simulink model "ieee_80211b_rx"  (R2018a)
settings: Solver=FixedStepDiscrete  StartTime=0.0  StopTime=length(rcvd.signals.values)*(p80211.SamplesPerChannelFrame / (p80211.ChipRate*p80211.SamplesPerChip))  RelTol=1e-3
InitFcn:
  | init;
  | load('data', 'rcvd');
model workspace: external: MAT-File (data not in the file)
values from neighbouring files (symbols this model uses):
  p80211 = commwlan80211BeaconRxInit(agcStepSize, agcMaxGain,      corrThreshold, sampsPerChip)    [wlan80211BeaconRxModelParams.m]
libraries: commwlan80211BeaconLib x3, commsync2 x2, dspsigops x2, commdigbbndpm3 x1, commsequence2 x1, dspnetwork x1, commrfcorlib x1, commfilt2 x1
Description:
  | IEEE 802.11 WLAN Beacon Frame Receiver for Captured Data
  | 
  | This example shows how to process a captured beacon frame and display the
  | frame information.
settings Model: Creator=The MathWorks, Inc.  LastModifiedBy=tung
settings DataIOCC: LimitDataPoints=on  SaveFormat=Array  SaveOutput=off  SignalLogging=off  DSMLogging=off  SaveTime=off
settings OptimizationCC: DefaultParameterBehavior=Inlined  InlineInvariantSignals=on  ExpressionDepthLimit=2147483647  EfficientFloat2IntCast=on  LifeSpan=inf
settings DebuggingCC: UnderspecifiedInitializationDetection=Classic  MergeDetectMultiDrivingBlocksExec=none  SolverPrmCheckMsg=warning  UniqueDataStoreMsg=error  AllowSymbolicDim=off  StateNameClashWarn=warning  SFUnexpectedBacktrackingDiag=warning  SFNoUnconditionalDefaultTransitionDiag=warning  SFExecutionAtInitializationDiag=none
settings HardwareCC: ProdBitPerPointer=32  ProdBitPerSizeT=32  ProdBitPerPtrDiffT=32  ProdLargestAtomicFloat=None  ProdIntDivRoundTo=Undefined  ProdEndianess=Unspecified  ProdWordSize=32  ProdHWDeviceType=32-bit Generic
settings ModelReferenceCC: PropagateSignalLabelsOutOfModel=off
settings CodeAppCC: StateflowObjectComments=on
settings GRTTargetCC: TargetLangStandard=C89/C90 (ANSI)  GeneratePreprocessorConditionals=Disable all  CombineOutputUpdateFcns=off  GRTInterface=on
settings ConfigComp: CovMetricSettings=dw  CovHtmlReporting=on  CovSaveCumulativeToWorkspaceVar=on  CovSaveSingleToWorkspaceVar=on  CovShowResultsExplorer=off  CovExternalEMLEnable=off  CovSFcnEnable=off

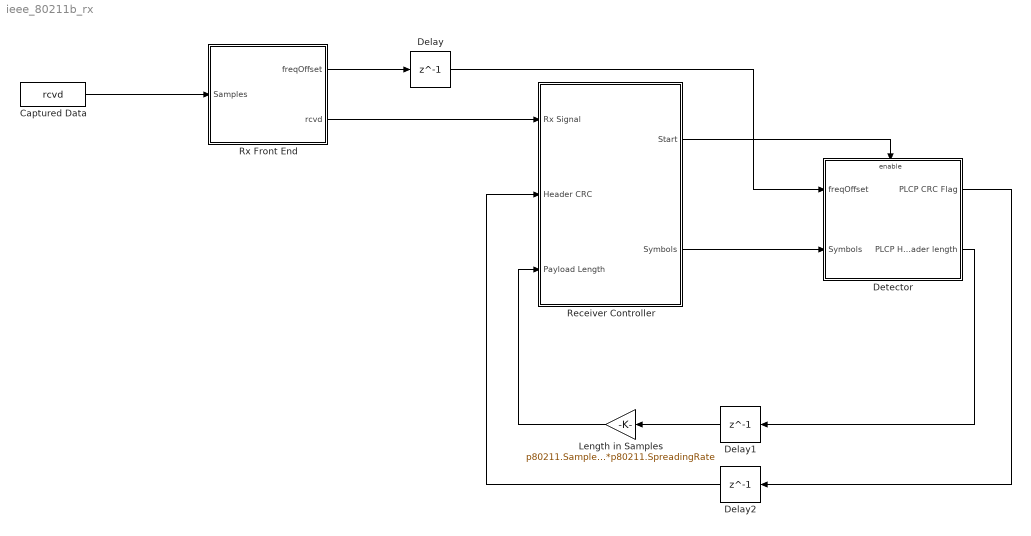
== system ieee_80211b_rx ==
  Captured Data : FromWorkspace  VariableName=rcvd  SampleTime=p80211.SamplesPerChannelFrame / (p80211.ChipRate*p80211.SamplesPerChip)  Interpolate=off  OutputAfterFinalValue=Cyclic repetition
  Delay : Delay  DelayLength=1  InitialCondition=0  InputProcessing=Columns as channels (frame based)
  Delay1 : Delay  DelayLength=1  InitialCondition=0  InputProcessing=Columns as channels (frame based)
  Delay2 : Delay  DelayLength=1  InitialCondition=0  InputProcessing=Columns as channels (frame based)
  Detector : Subsystem
      settings: CloseFcn=clear BeaconFrameBodyType rcvd
  Length in Samples : Gain  Gain=p80211.SamplesPerChip*p80211.SpreadingRate  OutDataTypeStr=uint32  SaturateOnIntegerOverflow=on  ParamDataTypeStr=Inherit: Same as input
  Receiver Controller : Subsystem
  Rx Front End : Subsystem
  wires:
  Length in Samples/1 -> Receiver Controller/3(Payload Length)
  Detector/1(PLCP CRC Flag) -> Delay2/1
  Delay2/1 -> Receiver Controller/2(Header CRC)
  Receiver Controller/1(Start) -> Detector/Enable
  Rx Front End/2(rcvd) -> Receiver Controller/1(Rx Signal)
  Delay1/1 -> Length in Samples/1
  Receiver Controller/2(Symbols) -> Detector/2(Symbols)
  Captured Data/1 -> Rx Front End/1(Samples)
  Detector/2(PLCP Header length) -> Delay1/1
  Rx Front End/1(freqOffset) -> Delay/1
  Delay/1 -> Detector/1(freqOffset)

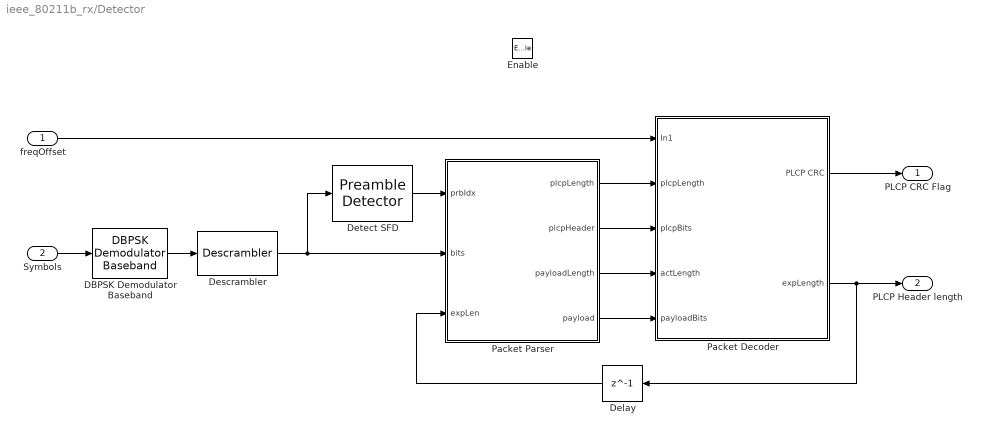
== system ieee_80211b_rx/Detector ==
  freqOffset : Inport
  Symbols : Inport  Port=2
  Enable : EnablePort  StatesWhenEnabling=reset  PropagateVarSize=During execution
  DBPSK Demodulator Baseband : commdigbbndpm3/DBPSK Demodulator Baseband  Ph=0  outDtype=Smallest unsigned integer
      settings: SourceProductName=Communications System Toolbox  SourceProductBaseCode=CM
  Delay : Delay  DelayLength=1  InitialCondition=0  InputProcessing=Columns as channels (frame based)
  Descrambler : commsequence2/Descrambler  M=2  poly=p80211.ScramblerPolynomial  iniStaSource=Dialog Parameter  ini_sta=[0 0 0 0 0 0 0]  resetViaPort=off
      settings: SourceProductName=Communications System Toolbox  SourceProductBaseCode=CM
  Detect SFD : commsync2/Preamble Detector  Input=Bit  Preamble=p80211.SFD  Threshold=3  DetectionMetricOutput=off  Detections=All  SimulateUsing=Code generation
      settings: SourceProductName=Communications System Toolbox  SourceProductBaseCode=CM
  Packet Decoder : Subsystem
  Packet Parser : MATLAB Function  TreatAsAtomicUnit=on
  PLCP CRC Flag : Outport  InitialOutput=1
  PLCP Header length : Outport  Port=2  InitialOutput=1
  wires:
  Delay/1 -> Packet Parser/3(expLen)
  Symbols/1 -> DBPSK Demodulator Baseband/1
  DBPSK Demodulator Baseband/1 -> Descrambler/1
  Detect SFD/1 -> Packet Parser/1(prbIdx)
  Descrambler/1 -> Detect SFD/1, Packet Parser/2(bits)
  Packet Decoder/1(PLCP CRC) -> PLCP CRC Flag/1
  Packet Decoder/2(expLength) -> Delay/1, PLCP Header length/1
  Packet Parser/1(plcpLength) -> Packet Decoder/2(plcpLength)
  Packet Parser/2(plcpHeader) -> Packet Decoder/3(plcpBits)
  Packet Parser/3(payloadLength) -> Packet Decoder/4(actLength)
  Packet Parser/4(payload) -> Packet Decoder/5(payloadBits)
  freqOffset/1 -> Packet Decoder/1(In1)

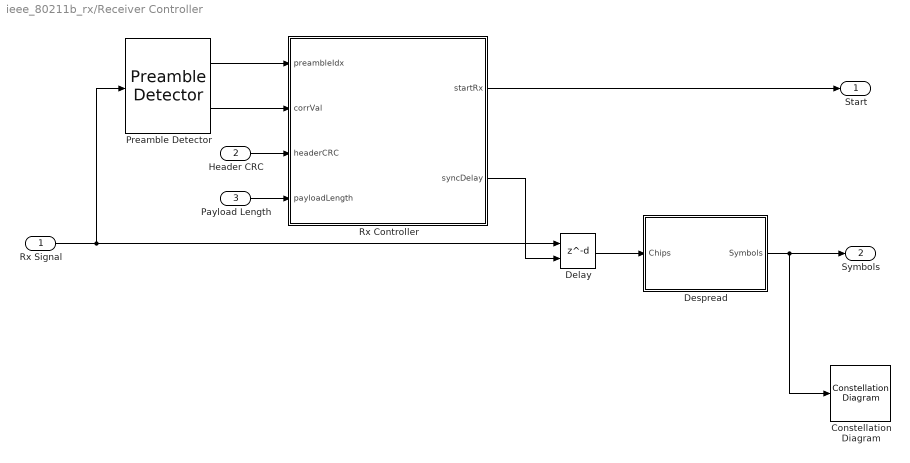
== system ieee_80211b_rx/Receiver Controller ==
  Rx Signal : Inport
  Header CRC : Inport  Port=2
  Payload Length : Inport  Port=3
  Constellation Diagram : ConstellationDiagram
  Delay : Delay  DelayLengthSource=Input port  DelayLengthUpperLimit=p80211.SamplesPerChannelFrame  InputProcessing=Columns as channels (frame based)
      settings: InputPortMap=u0,p1
  Despread : Subsystem
  Preamble Detector : commsync2/Preamble Detector  Input=Symbol  Preamble=p80211.SynchronizationSignal  Threshold=p80211.CorrelationThreshold  DetectionMetricOutput=on  Detections=All  SimulateUsing=Code generation
      settings: SourceProductName=Communications System Toolbox  SourceProductBaseCode=CM
  Rx Controller : MATLAB Function  TreatAsAtomicUnit=on
  Start : Outport
  Symbols : Outport  Port=2
  wires:
  Despread/1(Symbols) -> Constellation Diagram/1, Symbols/1
  Rx Controller/2(syncDelay) -> Delay/2
  Rx Controller/1(startRx) -> Start/1
  Header CRC/1 -> Rx Controller/3(headerCRC)
  Rx Signal/1 -> Preamble Detector/1, Delay/1
  Payload Length/1 -> Rx Controller/4(payloadLength)
  Delay/1 -> Despread/1(Chips)
  Preamble Detector/2 -> Rx Controller/2(corrVal)
  Preamble Detector/1 -> Rx Controller/1(preambleIdx)

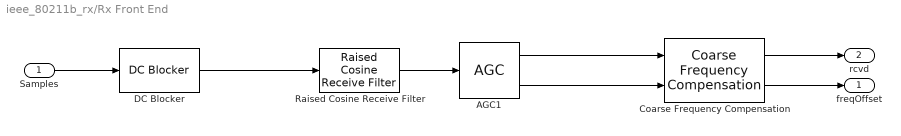
== system ieee_80211b_rx/Rx Front End ==
  Samples : Inport
  AGC1 : commrfcorlib/AGC  LegacyMode=off  DetectorMethod=Rectifier  LoopMethod=Linear  UpdatePeriod=100  StepSize=0.1  AdaptationStepSize=p80211.AGCStepSize  DesiredOutputPower=1  AveragingLength=50  MaximumGain=30  MaxPowerGain=p80211.AGCUpperLimit  GainOutputPort=off  InputPowerOutputPort=on  SimulateUsing=Code generation
      settings: SourceProductName=Communications System Toolbox
  Coarse Frequency Compensation : commwlan80211BeaconLib/Coarse Frequency Compensation  decimRate=44*p80211.SamplesPerChip/2  maxOffset=50000  M=2
      settings: SourceProductName=Communications System Toolbox  SourceProductBaseCode=CM
  DC Blocker : dspsigops/DC Blocker  Algorithm=IIR  NormalizedBandwidth=0.001  Length=8  Order=6  SimulateUsing=Code generation
      settings: SourceProductName=DSP System Toolbox  SourceProductBaseCode=DS
  Raised Cosine Receive Filter : commfilt2/Raised Cosine Receive Filter  filtType=Square root  R=0.3  filtSpan=p80211.FilterOrder  N=p80211.SamplesPerChip  downFactor=1  downOffset=0  filterGain=1  InputProcessing=Columns as channels (frame based)  RateOptions=Enforce single-rate processing  framing=Mute  checkCoeff=off  variableName=rcRxFilt  currentFiltSpan=2*(p80211.FilterOrder/2)  D=p80211.FilterOrder/2  inputOffset=0  sampMode=Mute  saveAsFlag=0  rateMode=Downsampling  checkGain=Normalized  launchFVT=off  roundingMode=Floor  overflowMode=off  coeffDataTypeStr=Inherit: Same word length as input  coeffMin=[]  coeffMax=[]  coeffLastDataTypeStr=Inherit: Same word length as input  accumDataTypeStr=Inherit: Same as product output  accumLastDataTypeStr=Inherit: Same as product output  outputDataTypeStr=Inherit: Same as accumulator  outputMin=[]  outputMax=[]  outputLastDataTypeStr=Inherit: Same as accumulator
  freqOffset : Outport
  rcvd : Outport  Port=2
  wires:
  Coarse Frequency Compensation/1 -> rcvd/1
  Samples/1 -> DC Blocker/1
  Raised Cosine Receive Filter/1 -> AGC1/1
  AGC1/1 -> Coarse Frequency Compensation/1
  AGC1/2 -> Coarse Frequency Compensation/2
  DC Blocker/1 -> Raised Cosine Receive Filter/1
  Coarse Frequency Compensation/2 -> freqOffset/1

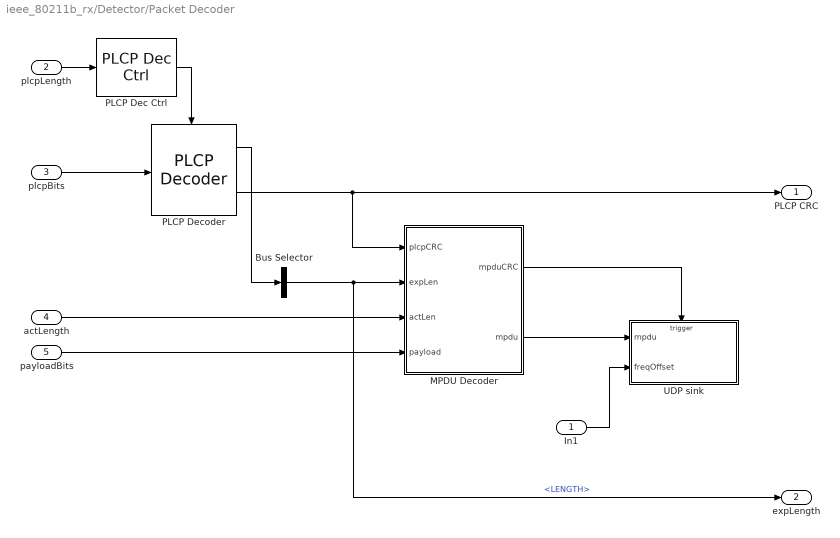
== system ieee_80211b_rx/Detector/Packet Decoder ==
  In1 : Inport
  plcpLength : Inport  Port=2
  plcpBits : Inport  Port=3
  actLength : Inport  Port=4
  payloadBits : Inport  Port=5
  Bus Selector : BusSelector  OutputSignals=LENGTH
  MPDU Decoder : MATLAB Function  TreatAsAtomicUnit=on
  PLCP Dec Ctrl : commwlan80211BeaconLib/Packet Decoder/PLCP Dec Ctrl
      settings: SourceProductName=Communications System Toolbox  SourceProductBaseCode=CM
  PLCP Decoder : commwlan80211BeaconLib/Packet Decoder/PLCP Decoder
      settings: SourceProductName=Communications System Toolbox  SourceProductBaseCode=CM
  UDP sink : Subsystem
  PLCP CRC : Outport
  expLength : Outport  Port=2
  wires:
  payloadBits/1 -> MPDU Decoder/4(payload)
  PLCP Dec Ctrl/1 -> PLCP Decoder/Trigger
  plcpBits/1 -> PLCP Decoder/1
  Bus Selector/1 -> MPDU Decoder/2(expLen), expLength/1  "<LENGTH>"
  actLength/1 -> MPDU Decoder/3(actLen)
  plcpLength/1 -> PLCP Dec Ctrl/1
  PLCP Decoder/2 -> PLCP CRC/1, MPDU Decoder/1(plcpCRC)
  PLCP Decoder/1 -> Bus Selector/1
  MPDU Decoder/1(mpduCRC) -> UDP sink/Trigger
  MPDU Decoder/2(mpdu) -> UDP sink/1(mpdu)
  In1/1 -> UDP sink/2(freqOffset)

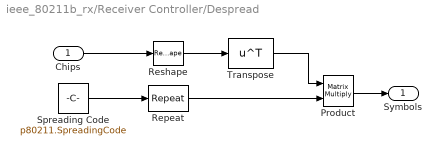
== system ieee_80211b_rx/Receiver Controller/Despread ==
  Chips : Inport
  Product : Product  Multiplication=Matrix(*)  RndMeth=Zero
  Repeat : dspsigops/Repeat  N=p80211.SamplesPerChip  InputProcessing=Columns as channels (frame based)  RateOptions=Enforce single-rate processing  ic=0  mode=Unused parameter value
      settings: SourceProductName=DSP System Toolbox
  Reshape : Reshape  OutputDimensionality=Customize  OutputDimensions=[length(p80211.SpreadingCode)*p80211.SamplesPerChip, p80211.SymbolsPerChannelFrame]
  Spreading Code : Constant  Value=p80211.SpreadingCode  VectorParams1D=off
  Transpose : Math  Operator=transpose  SaturateOnIntegerOverflow=on
  Symbols : Outport
  wires:
  Transpose/1 -> Product/1
  Repeat/1 -> Product/2
  Reshape/1 -> Transpose/1
  Chips/1 -> Reshape/1
  Product/1 -> Symbols/1
  Spreading Code/1 -> Repeat/1

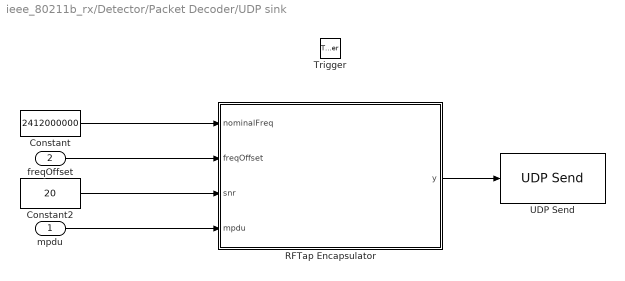
== system ieee_80211b_rx/Detector/Packet Decoder/UDP sink ==
  mpdu : Inport
  freqOffset : Inport  Port=2
  Trigger : TriggerPort  TriggerType=falling  VariantControl=Variant  PortDimensions=1
  Constant : Constant  Value=2412000000
  Constant2 : Constant  Value=20  OutDataTypeStr=single
  RFTap Encapsulator : MATLAB Function  TreatAsAtomicUnit=on
  UDP Send : dspnetwork/UDP Send  remoteURL='127.0.0.1'  remotePort=25000  localURL='0.0.0.0'  localPortSource=Automatically determine  localPort=-1  sampletime=-1  blockPlatform=[]  separateLengthPort=0
      settings: SourceProductName=DSP System Toolbox  SourceProductBaseCode=DS
  wires:
  RFTap Encapsulator/1(y) -> UDP Send/1
  mpdu/1 -> RFTap Encapsulator/4(mpdu)
  Constant/1 -> RFTap Encapsulator/1(nominalFreq)
  freqOffset/1 -> RFTap Encapsulator/2(freqOffset)
  Constant2/1 -> RFTap Encapsulator/3(snr)

== matlab function ieee_80211b_rx/Detector/Packet Parser ==
  data: prbIdx input; plcpLength output; plcpHeader output size=[p80211.PLCPHeaderLength 1]; payloadLength output; bits input; expLen input; p80211 parameter; payload output size=[p80211.PayloadBufferLength 1]
function [plcpLength, plcpHeader, payloadLength, payload] = ...
  parsePacket(prbIdx, bits, expLen, p80211)

%#codegen

persistent plcpCount payloadCount plcpBuffer payloadBuffer controllerState

% State enums
SearchSFD      = 0;
ReceivePLCP    = 1;
ReceivePayload = 2;


if isempty(plcpCount)
  plcpCount = uint16(1);
  payloadCount = uint16(1);
  % 8 extra bits for synchronizing descrambler
  plcpBuffer = false(p80211.PLCPHeaderLength, 1);
  payloadBuffer = false(p80211.PayloadBufferLength, 1);
  controllerState = SearchSFD;
end

inputLen = uint16(length(bits));
plcpBufferLen = uint16(length(plcpBuffer));
payloadLength = uint16(1);

switch controllerState
  case SearchSFD
    if ~isempty(prbIdx)
      preambleIdx = prbIdx(1);  
      numPLCPBits = inputLen-preambleIdx-1;
      if numPLCPBits >= plcpBufferLen
        plcpBuffer(:) = bits(preambleIdx+(1:plcpBufferLen));
        plcpCount = plcpCount + plcpBufferLen;
        payloadBuffer(1:inputLen-plcpBufferLen-preambleIdx) = ...
          bits(plcpBufferLen+preambleIdx+1:end);
        controllerState = ReceivePayload;
        payloadCount = inputLen-plcpBufferLen-preambleIdx+1;
      else
        plcpBuffer(1:numPLCPBits) = bits(preambleIdx+(1:numPLCPBits));
        plcpCount = plcpCount + numPLCPBits;
        controllerState = ReceivePLCP;
      end
    end
  case ReceivePLCP
    plcpLen = p80211.PLCPHeaderLength;
    if (plcpCount + inputLen) < plcpLen
      plcpBuffer(plcpCount + (1:inputLen)) = bits;
      plcpCount = plcpCount + inputLen;
    else
      plcpBuffer(plcpCount:end) = bits(1:plcpLen-plcpCount+1);
      payloadBuffer(1:inputLen-(plcpLen-plcpCount+1)) = ...
        bits(plcpLen-plcpCount+2:end);
      controllerState = ReceivePayload;
    end
  case ReceivePayload
    payloadBuffer(payloadCount+(0:inputLen-1)) = bits;
    payloadCount = payloadCount + inputLen;
    payloadLength = payloadCount - 1;
    if payloadCount > expLen
      controllerState = SearchSFD;
      plcpCount = uint16(1);
      payloadCount = uint16(1);
    end
end

plcpLength = plcpCount - 1;
plcpHeader = plcpBuffer;
payload = payloadBuffer;

== matlab function ieee_80211b_rx/Detector/Packet Decoder/MPDU Decoder ==
  data: plcpCRC input; mpduCRC output; expLen input; actLen input; payload input; mpdu output size=[p80211.PayloadBufferLength-32 1]
function [mpduCRC, mpdu] = mpduDecode(plcpCRC, expLen, actLen, payload)
%#codegen

persistent hCRC firstTime lastMPDU lastMpduCRC

% Frame check sequence (FCS)
if isempty(hCRC)
    hCRC = comm.CRCDetector([32 26 23 22 16 12 11 10 8 7 5 4 2 1 0], ...
        'InitialConditions', 1, ...
        'DirectMethod',      true, ...
        'FinalXOR',          1);
    firstTime = true;
    lastMPDU = false(length(payload)-32, 1);
    lastMpduCRC = true;  % CRC is not zero
end

% If the CRC for the header decodes correctly (i.e. CRC flag is 0) and the
% received MPDU payload length is greater than or equal to the expected
% length, then turn on the MPDU decoder
if ~plcpCRC && (expLen > 0) && (actLen >= expLen) && (expLen >= 32) ...
        && firstTime
    % Compute CRC based on IEEE Std 802.11(TM)-2007 section 7.1.3.7.
    frameCRC = payload(1:expLen);
    [t1, t2] = step(hCRC, frameCRC);
    mpdu = logical(t1);
    mpduCRC = logical(t2);
    lastMPDU(1:expLen-32) = mpdu;
    lastMPDU(expLen-31:end) = false;
    lastMpduCRC = mpduCRC;
    firstTime = false;
else
    mpdu = lastMPDU;
    mpduCRC = lastMpduCRC;
end

== matlab function ieee_80211b_rx/Receiver Controller/Rx Controller ==
  data: preambleIdx input; corrVal input; startRx output; headerCRC input boolean size=[1 1]; payloadLength input size=1; p80211 parameter; syncDelay output
function [startRx, syncDelay] = ...
  rxCtrl(preambleIdx, corrVal, headerCRC, payloadLength, p80211)
%#codegen

persistent rxOn controllerState payloadCount lastSyncDelay corrPeakValOld

% State Enums
SearchPLCP = 0;
GetPLCP    = 2;
GetPayload = 4;

if isempty(rxOn)
  % Initialize receiver controller
  rxOn = false;
  controllerState = SearchPLCP;
  payloadCount = 0;
  lastSyncDelay = 0;
  corrPeakValOld = 0;
end

if isempty(preambleIdx)
    corrPeakVal = 0;
    preambleDetected = false;
else
    corrPeakVal = corrVal(preambleIdx(1));
    preambleDetected = true;
end

if (corrPeakValOld < corrPeakVal)
  controllerState = SearchPLCP;
end

switch controllerState
  case SearchPLCP
    % Search for the PLCP SYNC signal
    
    if preambleDetected
      corrPeakValOld = corrPeakVal;
      % Synchronize to the end of the SYNC. Get 8 (scrambler length) extra
      % bits to initialize DPSK demodulator and scrambler
      scramblerLen = length(p80211.ScramblerPolynomial);
      lastSyncDelay = p80211.SamplesPerChannelFrame - (preambleIdx(1) ...
        - scramblerLen*p80211.SpreadingRate*p80211.SamplesPerChip); 
      payloadCount = p80211.NumSYNCSamples ...
        - scramblerLen*p80211.SpreadingRate*p80211.SamplesPerChip;
      rxOn = true;
      
      controllerState = GetPLCP;
    end
  case GetPLCP
    % In this state we receive both SFD, which is part of PLCP preamble,
    % and the PLCP header
    
    payloadCount = payloadCount + p80211.SamplesPerChannelFrame;
    
    if (payloadCount >= ...
        (p80211.NumPLCPSamples+p80211.ScramblerAmbiguitySamples))
    % Wait one more channel frame to let the PLCP CRC result to reach.
    % There is a delay between detector and receiver controller to break
    % the algebraic loop.
      if headerCRC ~= 1
        controllerState = GetPayload;
      else
        rxOn = false;
        lastSyncDelay = 0;
        payloadCount = 0;
        controllerState = SearchPLCP;
      end
    end
  case GetPayload
    % Receive payload symbols
    
    payloadCount = payloadCount + p80211.SamplesPerChannelFrame;
    
    if payloadCount >= ...
        ((p80211.NumPLCPSamples+p80211.ScramblerAmbiguitySamples) + ...
        payloadLength)
      rxOn = false;
      lastSyncDelay = 0;
      payloadCount = 0;
      controllerState = SearchPLCP;
    end
end

startRx = rxOn;
syncDelay = lastSyncDelay;

== matlab function ieee_80211b_rx/Detector/Packet Decoder/UDP sink/RFTap Encapsulator ==
  data: nominalFreq input; freqOffset input; snr input single; mpdu input size=[p80211.PayloadBufferLength-32 1]; y output size=[(p80211.PayloadBufferLength-32)/8+32 1]
function y = rftapEncapsulate(nominalFreq, freqOffset, snr, mpdu)

uiHeader        = uint8(hex2dec(['52'; '46'; '74'; '61'; '08'; '00'; '8d'; '00']));
uiDatalinkType  = uint8(hex2dec(['69'; '00'; '00'; '00']));
uiNominalFreq   = uint8(flipud(hex2dec(reshape(num2hex(nominalFreq), 2, []).')));
uiFreqOffset    = uint8(flipud(hex2dec(reshape(num2hex(freqOffset) , 2, []).')));
uiSNR           = uint8(flipud(hex2dec(reshape(num2hex(snr)        , 2, []).')));
uiMpdu          = uint8(bi2de(reshape(mpdu, 8, []).', 'right-msb'));

y = [uiHeader; uiDatalinkType; uiNominalFreq; uiFreqOffset; uiSNR; uiMpdu];
